simulink model "Case3AtLoad100"  (R2023b)
settings: Solver=VariableStepAuto  StartTime=0.0  StopTime=10  RelTol=1e-3
libraries: spsSeriesRLCBranchLib x15, spsRMSLib x4, spsCurrentMeasurementLib x2, spsVoltageMeasurementLib x2, spsACVoltageSourceLib x1, spsGroundLib x1, spsPowerLib x1, sps_lib x1
settings Model: Creator=ASUS  LastModifiedBy=ASUS

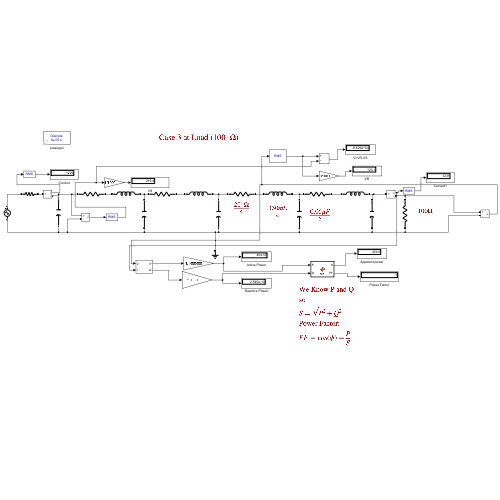
[thumbnail: Simulink's stored preview of the top-level diagram]
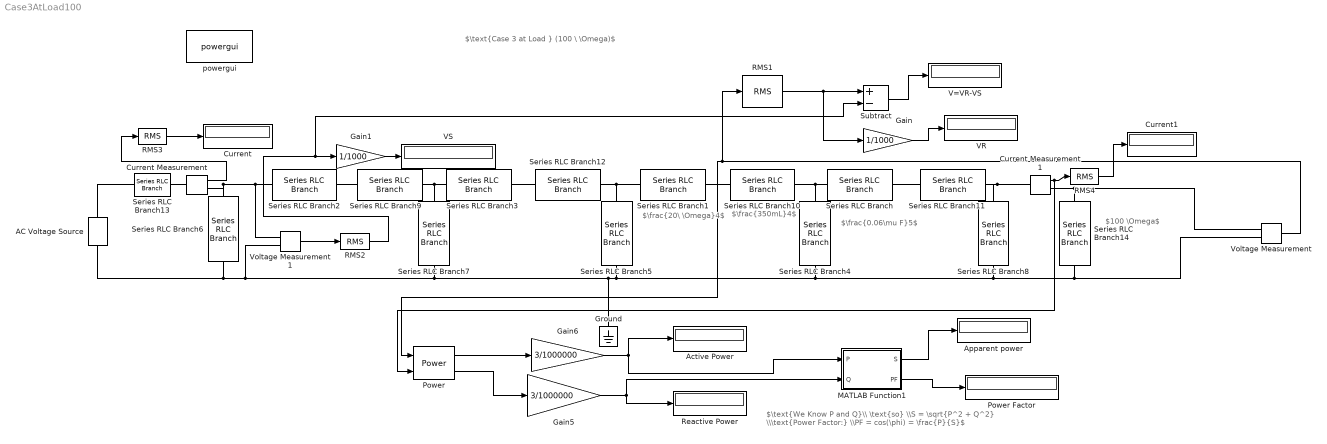
== system Case3AtLoad100 ==
  note: $\text{We Know P and Q}\\ \text{so} \\S = \sqrt{P^2 + Q^2} \\\text{Power Factor:} \\PF = cos(\phi) = \frac{P}{S}$
  note: $\text{Case 3 at Load } (100 \ \Omega)$
  note: $\frac{20\ \Omega}4$
  note: $\frac{350mL}4$
  note: $\frac{0.06\mu F}5$
  note: $100 \Omega$
  AC Voltage Source : spsACVoltageSourceLib/AC Voltage Source  Amplitude=sqrt(2)*(380e3/sqrt(3))  Phase=0  Frequency=60  SampleTime=50e-6  Measurements=None  BusType=swing  Pref=10e3  Qref=0  Qmin=-inf  Qmax=+inf
  Active Power : Display
      settings: Format=bank
  Apparent power : Display
  Current : Display
  Current Measurement : spsCurrentMeasurementLib/Current Measurement  PhasorSimulation=off  OutputType=Complex  PSBequivalent=0
  Current Measurement1 : spsCurrentMeasurementLib/Current Measurement  PhasorSimulation=off  OutputType=Complex  PSBequivalent=0
  Current1 : Display
  Gain : Gain  Gain=1/1000
  Gain1 : Gain  Gain=1/1000
  Gain5 : Gain  Gain=3/1000000
  Gain6 : Gain  Gain=3/1000000
  Ground : spsGroundLib/Ground  LConnTagsString=a
  MATLAB Function1 : MATLAB Function  TreatAsAtomicUnit=on
  Power : spsPowerLib/Power  Freq=60  Vinit=[1, 0]  Iinit=[1, 0]  Ts=50e-6
  Power Factor : Display
  RMS{1..4} (4 alike) : spsRMSLib/RMS  TrueRMS=on  Freq=60  RMSInit=0  Ts=0
  Reactive Power : Display
  Series RLC Branch{,1..3} (4 alike) : spsSeriesRLCBranchLib/Series RLC Branch  LConnTagsString=__new0  RConnTagsString=__new0  BranchType=R  Resistance=20/4  Inductance=1e-3  SetiL0=off  InitialCurrent=0  Capacitance=1e-6  Setx0=off  InitialVoltage=0  Measurements=None
  Series RLC Branch{9..12} (4 alike) : spsSeriesRLCBranchLib/Series RLC Branch  LConnTagsString=__new0  RConnTagsString=__new0  BranchType=L  Resistance=350e-3/4  Inductance=350e-3/4  SetiL0=off  InitialCurrent=0  Capacitance=0.06e-6/4  Setx0=off  InitialVoltage=0  Measurements=None
  Series RLC Branch13 : spsSeriesRLCBranchLib/Series RLC Branch  LConnTagsString=__new0  RConnTagsString=__new0  BranchType=R  Resistance=0.001  Inductance=1e-3  SetiL0=off  InitialCurrent=0  Capacitance=1e-6  Setx0=off  InitialVoltage=0  Measurements=None
  Series RLC Branch14 : spsSeriesRLCBranchLib/Series RLC Branch  LConnTagsString=__new0  RConnTagsString=__new0  BranchType=R  Resistance=100  Inductance=1e-3  SetiL0=off  InitialCurrent=0  Capacitance=1e-6  Setx0=off  InitialVoltage=0  Measurements=None
  Series RLC Branch{4..5,7..8} (4 alike) : spsSeriesRLCBranchLib/Series RLC Branch  LConnTagsString=__new0  RConnTagsString=__new0  BranchType=C  Resistance=20/4  Inductance=1e-3  SetiL0=off  InitialCurrent=0  Capacitance=0.06e-6/5  Setx0=off  InitialVoltage=0  Measurements=None
  Series RLC Branch6 : spsSeriesRLCBranchLib/Series RLC Branch  LConnTagsString=__new0  RConnTagsString=__new0  BranchType=C  Resistance=20/4  Inductance=1e-3  SetiL0=off  InitialCurrent=0  Capacitance=0.04e-6/5  Setx0=off  InitialVoltage=0  Measurements=None
  Subtract : Sum  Inputs=+-
  V=VR-VS : Display
  VR : Display
  VS : Display
  Voltage Measurement : spsVoltageMeasurementLib/Voltage Measurement  PhasorSimulation=off  OutputType=Complex  PSBequivalent=0
  Voltage Measurement1 : spsVoltageMeasurementLib/Voltage Measurement  PhasorSimulation=off  OutputType=Complex  PSBequivalent=0
  powergui : sps_lib/powergui  Priority=1  SimulationMode=Discrete  SampleTime=50e-6  frequency=60  Iterations=50  frequencyindice=60  Pbase=100e6  ErrMax=1e-4  UnitsV=kV  UnitsW=MW  buscounter=0  FunctionMessages=off  echomessages=off  EnableUseOfTLC=off  CurrentSourceSwitches=off  DisableSnubberDevices=off  DisableRonSwitches=off  DisableVfSwitches=off  DisplayEquations=off  AutomaticDiscreteSolvers=off  SolverType=Tustin/Backward Euler (TBE)  Interpol=off  ExternalGateDelay=off  methode=off  Ts=100  x0status=blocks  SPID=on  SwTol=0  HookPort=off  NonlinearTolerance=1e-4  nMaxIteration=100  ContinueOnMaxIteration=off  RestoreLinks=warning  ResistiveCurrentMeasurement=off  Frange=[0:2:500]  Ylog=off  Xlog=on  ShowGrid=off  save=off  variable=ZData  structure=0  ZoomFFT=off  StartTime=0.0  cycles=1  DisplayStyle=1  fundamental=60  FreqAxis=off  MaxFrequency=1000  frequencyindicesteady=1  RmsSteady=1  display=off
  wires:
  Voltage Measurement1/1 -> RMS2/1
  Gain/1 -> VR/1
  Gain1/1 -> VS/1
  Current Measurement/1 -> RMS3/1
  RMS3/1 -> Current/1
  RMS2/1 -> Subtract/2, Gain1/1
  Power/2 -> Gain5/1
  Power/1 -> Gain6/1
  Gain6/1 -> Active Power/1, MATLAB Function1/1(P)
  Gain5/1 -> Reactive Power/1, MATLAB Function1/2(Q)
  MATLAB Function1/1(S) -> Apparent power/1
  MATLAB Function1/2(PF) -> Power Factor/1
  Subtract/1 -> V=VR-VS/1
  RMS1/1 -> Gain/1, Subtract/1
  Voltage Measurement/1 -> Power/1, RMS1/1
  Current Measurement1/1 -> Power/2, RMS4/1
  RMS4/1 -> Current1/1
  connections:
  Series RLC Branch2/RConn1 -- Series RLC Branch9/LConn1
  Series RLC Branch12/LConn1 -- Series RLC Branch3/RConn1
  Series RLC Branch12/RConn1 -- Series RLC Branch5/LConn1 -- Series RLC Branch1/LConn1
  Series RLC Branch1/RConn1 -- Series RLC Branch10/LConn1
  Series RLC Branch11/LConn1 -- Series RLC Branch/RConn1
  Series RLC Branch/LConn1 -- Series RLC Branch10/RConn1 -- Series RLC Branch4/LConn1
  Series RLC Branch11/RConn1 -- Series RLC Branch8/LConn1 -- Current Measurement1/LConn1
  Series RLC Branch8/RConn1 -- Voltage Measurement/LConn2 -- Series RLC Branch14/RConn1 -- Series RLC Branch4/RConn1 -- Ground/LConn1 -- Series RLC Branch6/RConn1 -- AC Voltage Source/LConn1 -- Voltage Measurement1/LConn2 -- Series RLC Branch7/RConn1 -- Series RLC Branch5/RConn1
  Series RLC Branch13/LConn1 -- AC Voltage Source/RConn1
  Series RLC Branch3/LConn1 -- Series RLC Branch7/LConn1 -- Series RLC Branch9/RConn1
  Current Measurement/LConn1 -- Series RLC Branch13/RConn1
  Series RLC Branch2/LConn1 -- Current Measurement/RConn1 -- Series RLC Branch6/LConn1 -- Voltage Measurement1/LConn1
  Series RLC Branch14/LConn1 -- Current Measurement1/RConn1 -- Voltage Measurement/LConn1

== matlab function Case3AtLoad100/MATLAB Function1 ==
  data: P input; S output; Q input; PF output
function [S,PF] = fcn(P,Q)
P=abs(P);
S=sqrt(Q^2+P^2);
PF=P/S;
